simulink model "adaptive3"  (Simulink 7.1)
settings: Solver=ode45  StartTime=0.0  StopTime=100  RelTol=1e-3
InitFcn:
  | vo=502;
  | za=-1.01887*502;
  | zq=0.0949*502;
  | zd=-0.00215*502;
  | ma=0.82225;
  | mq=-1.07741;
  | md=-0.17555;
settings Model: Creator=Yaghobi  LastModifiedBy=Yaghobi

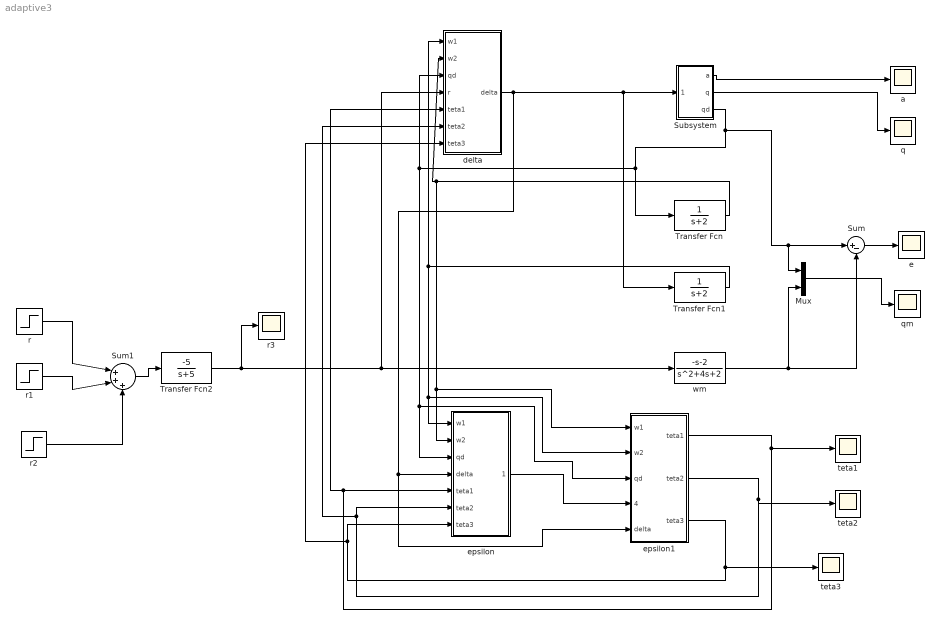
== system adaptive3 ==
  Mux : Mux  Inputs=2
  Subsystem : Subsystem
  Sum : Sum  Inputs=|+-  OutDataType=sfix(16)  OutScaling=2^0
  Sum1 : Sum  Inputs=|+++  OutDataType=sfix(16)  OutScaling=2^0
  Transfer Fcn : TransferFcn  Denominator=[1 2]
  Transfer Fcn1 : TransferFcn  Denominator=[1 2]
  Transfer Fcn2 : TransferFcn  Numerator=[-5]  Denominator=[1 5]
  a : Scope
  delta : Subsystem
  e : Scope
      settings: SaveName=ScopeData6
  epsilon : Subsystem
  epsilon1 : Subsystem
  q : Scope
  qm : Scope
      settings: SaveName=q1  DataFormat=Array  MaxDataPoints=500000
  r : Step  Time=0  After=-1  SampleTime=0
  r1 : Step  Time=20  After=3  SampleTime=0
  r2 : Step  Time=40  After=-6  SampleTime=0
  r3 : Scope
      settings: SaveName=ScopeData7
  teta1 : Scope
      settings: SaveName=ScopeData3
  teta2 : Scope
      settings: SaveName=ScopeData4
  teta3 : Scope
      settings: SaveName=ScopeData5
  wm : TransferFcn  Numerator=[-1 -2]  Denominator="[1 4  2]"
  wires:
  Subsystem/1(a) -> a/1
  Subsystem/2(q) -> q/1
  Subsystem/3(qd) -> Transfer Fcn/1, delta/3(qd), epsilon/3(qd), epsilon1/3(qd), Sum/1, Mux/1
  delta/1(delta) -> Subsystem/1(delta), Transfer Fcn1/1, epsilon/4(delta), epsilon1/5(delta)
  wm/1 -> Sum/2, Mux/2
  Transfer Fcn/1 -> delta/2(w2), epsilon/2(w2), epsilon1/1(w1)
  Transfer Fcn1/1 -> delta/1(w1), epsilon/1(w1), epsilon1/2(w2)
  epsilon/1(epsilon) -> epsilon1/4(epsilon)
  epsilon1/1(teta1) -> epsilon/5(teta1), delta/5(teta1), teta1/1
  epsilon1/2(teta2) -> epsilon/6(teta2), delta/6(teta2), teta2/1
  epsilon1/3(teta3) -> epsilon/7(teta3), delta/7(teta3), teta3/1
  Sum/1 -> e/1
  r/1 -> Sum1/1
  r1/1 -> Sum1/2
  r2/1 -> Sum1/3
  Sum1/1 -> Transfer Fcn2/1
  Transfer Fcn2/1 -> wm/1, delta/4(r), r3/1
  Mux/1 -> qm/1

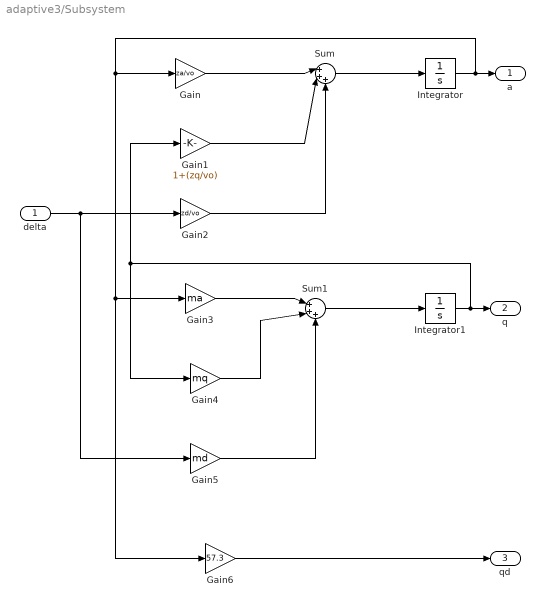
== system adaptive3/Subsystem ==
  delta : Inport
  Gain : Gain  Gain=za/vo  ParameterDataType=sfix(16)  ParameterScaling=2^0  OutDataType=sfix(16)  OutScaling=2^0
  Gain1 : Gain  Gain=1+(zq/vo)  ParameterDataType=sfix(16)  ParameterScaling=2^0  OutDataType=sfix(16)  OutScaling=2^0
  Gain2 : Gain  Gain=zd/vo  ParameterDataType=sfix(16)  ParameterScaling=2^0  OutDataType=sfix(16)  OutScaling=2^0
  Gain3 : Gain  Gain=ma  ParameterDataType=sfix(16)  ParameterScaling=2^0  OutDataType=sfix(16)  OutScaling=2^0
  Gain4 : Gain  Gain=mq  ParameterDataType=sfix(16)  ParameterScaling=2^0  OutDataType=sfix(16)  OutScaling=2^0
  Gain5 : Gain  Gain=md  ParameterDataType=sfix(16)  ParameterScaling=2^0  OutDataType=sfix(16)  OutScaling=2^0
  Gain6 : Gain  Gain=57.3  ParameterDataType=sfix(16)  ParameterScaling=2^0  OutDataType=sfix(16)  OutScaling=2^0
  Integrator : Integrator
  Integrator1 : Integrator
  Sum : Sum  Inputs=|+++  OutDataType=sfix(16)  OutScaling=2^0
  Sum1 : Sum  Inputs=|+++  OutDataType=sfix(16)  OutScaling=2^0
  a : Outport
  q : Outport  Port=2
  qd : Outport  Port=3
  wires:
  Integrator/1 -> Gain/1, Gain3/1, Gain6/1, a/1
  Gain/1 -> Sum/1
  Gain1/1 -> Sum/2
  Gain2/1 -> Sum/3
  Sum/1 -> Integrator/1
  Gain3/1 -> Sum1/1
  Gain4/1 -> Sum1/2
  Sum1/1 -> Integrator1/1
  Integrator1/1 -> Gain4/1, Gain1/1, q/1
  Gain5/1 -> Sum1/3
  delta/1 -> Gain2/1, Gain5/1
  Gain6/1 -> qd/1

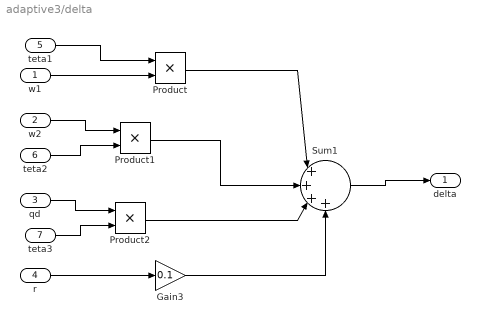
== system adaptive3/delta ==
  w1 : Inport
  w2 : Inport  Port=2
  qd : Inport  Port=3
  r : Inport  Port=4
  teta1 : Inport  Port=5
  teta2 : Inport  Port=6
  teta3 : Inport  Port=7
  Gain3 : Gain  Gain=0.1  ParameterDataType=sfix(16)  ParameterScaling=2^0  OutDataType=sfix(16)  OutScaling=2^0
  Product : Product  OutDataType=sfix(16)  OutScaling=2^0  RndMeth=Zero
  Product1 : Product  OutDataType=sfix(16)  OutScaling=2^0  RndMeth=Zero
  Product2 : Product  OutDataType=sfix(16)  OutScaling=2^0  RndMeth=Zero
  Sum1 : Sum  Inputs=|++++  OutDataType=sfix(16)  OutScaling=2^0
  delta : Outport
  wires:
  w1/1 -> Product/2
  r/1 -> Gain3/1
  teta1/1 -> Product/1
  w2/1 -> Product1/1
  teta2/1 -> Product1/2
  qd/1 -> Product2/1
  teta3/1 -> Product2/2
  Product/1 -> Sum1/1
  Product1/1 -> Sum1/2
  Product2/1 -> Sum1/3
  Gain3/1 -> Sum1/4
  Sum1/1 -> delta/1

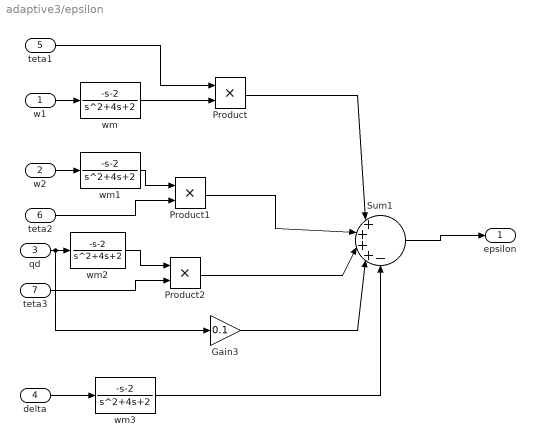
== system adaptive3/epsilon ==
  w1 : Inport
  w2 : Inport  Port=2
  qd : Inport  Port=3
  delta : Inport  Port=4
  teta1 : Inport  Port=5
  teta2 : Inport  Port=6
  teta3 : Inport  Port=7
  Gain3 : Gain  Gain=0.1  ParameterDataType=sfix(16)  ParameterScaling=2^0  OutDataType=sfix(16)  OutScaling=2^0
  Product : Product  OutDataType=sfix(16)  OutScaling=2^0  RndMeth=Zero
  Product1 : Product  OutDataType=sfix(16)  OutScaling=2^0  RndMeth=Zero
  Product2 : Product  OutDataType=sfix(16)  OutScaling=2^0  RndMeth=Zero
  Sum1 : Sum  Inputs=|++++-  OutDataType=sfix(16)  OutScaling=2^0
  wm{,1..3} (4 alike) : TransferFcn  Numerator=[-1 -2]  Denominator="[1 4  2]"
  epsilon : Outport
  wires:
  w1/1 -> wm/1
  teta1/1 -> Product/1
  w2/1 -> wm1/1
  teta2/1 -> Product1/2
  qd/1 -> wm2/1, Gain3/1
  teta3/1 -> Product2/2
  Product/1 -> Sum1/1
  Product1/1 -> Sum1/2
  Product2/1 -> Sum1/3
  Gain3/1 -> Sum1/4
  Sum1/1 -> epsilon/1
  wm/1 -> Product/2
  wm1/1 -> Product1/1
  wm2/1 -> Product2/1
  delta/1 -> wm3/1
  wm3/1 -> Sum1/5

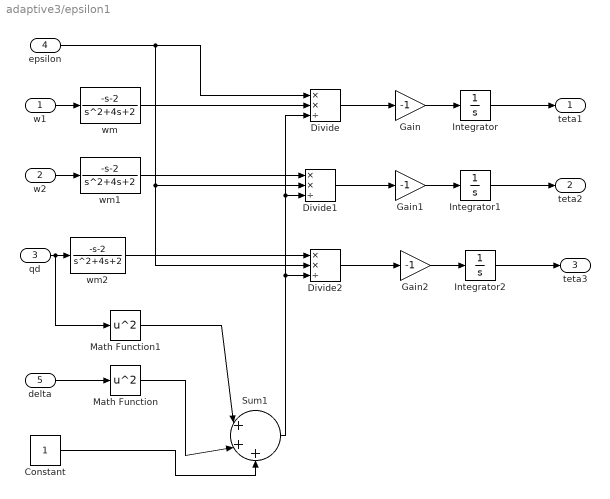
== system adaptive3/epsilon1 ==
  w1 : Inport
  w2 : Inport  Port=2
  qd : Inport  Port=3
  epsilon : Inport  Port=4
  delta : Inport  Port=5
  Constant : Constant  OutDataType=sfix(16)  OutScaling=2^0
  Divide : Product  Inputs=**/  OutDataType=sfix(16)  OutScaling=2^-10
  Divide1 : Product  Inputs=**/  OutDataType=sfix(16)  OutScaling=2^-10
  Divide2 : Product  Inputs=**/  OutDataType=sfix(16)  OutScaling=2^-10
  Gain : Gain  Gain=-1  ParameterDataType=sfix(16)  ParameterScaling=2^0  OutDataType=sfix(16)  OutScaling=2^0
  Gain1 : Gain  Gain=-1  ParameterDataType=sfix(16)  ParameterScaling=2^0  OutDataType=sfix(16)  OutScaling=2^0
  Gain2 : Gain  Gain=-1  ParameterDataType=sfix(16)  ParameterScaling=2^0  OutDataType=sfix(16)  OutScaling=2^0
  Integrator : Integrator  InitialCondition=1
  Integrator1 : Integrator  InitialCondition=.1
  Integrator2 : Integrator
  Math Function : Math  Operator=square  OutDataType=sfix(16)  OutScaling=2^0  SaturateOnIntegerOverflow=on
  Math Function1 : Math  Operator=square  OutDataType=sfix(16)  OutScaling=2^0  SaturateOnIntegerOverflow=on
  Sum1 : Sum  Inputs=|+++  OutDataType=sfix(16)  OutScaling=2^0
  wm : TransferFcn  Numerator=[-1 -2]  Denominator="[1 4  2]"
  wm1 : TransferFcn  Numerator=[-1 -2]  Denominator="[1 4  2]"
  wm2 : TransferFcn  Numerator=[-1 -2]  Denominator="[1 4  2]"
  teta1 : Outport
  teta2 : Outport  Port=2
  teta3 : Outport  Port=3
  wires:
  w1/1 -> wm/1
  w2/1 -> wm1/1
  qd/1 -> wm2/1, Math Function1/1
  wm/1 -> Divide/2
  wm1/1 -> Divide1/1
  wm2/1 -> Divide2/1
  epsilon/1 -> Divide/1, Divide1/2, Divide2/2
  delta/1 -> Math Function/1
  Math Function1/1 -> Sum1/1
  Math Function/1 -> Sum1/2
  Constant/1 -> Sum1/3
  Sum1/1 -> Divide/3, Divide1/3, Divide2/3
  Divide/1 -> Gain/1
  Gain/1 -> Integrator/1
  Integrator/1 -> teta1/1
  Divide1/1 -> Gain1/1
  Gain1/1 -> Integrator1/1
  Integrator1/1 -> teta2/1
  Divide2/1 -> Gain2/1
  Gain2/1 -> Integrator2/1
  Integrator2/1 -> teta3/1
